simulink subsystem "PvtSubSys_VSM_LCK"  (R2020b)
settings: Solver=VariableStepAuto  StartTime=0.0  StopTime=10.0  RelTol=1e-3
values from neighbouring files (symbols this model uses):
  LCK_STATE : value not decoded    [LCK.sldd]
  P_VSM_LCK_A1 = 15.0    [LCK.sldd]
  P_VSM_LCK_AbsEspInTime = 3.0    [LCK.sldd]
  P_VSM_LCK_absLongitudeAccIn = 2.5    [LCK.sldd]
  P_VSM_LCK_absLongitudeAccOut = 3.0    [LCK.sldd]
  P_VSM_LCK_AccRateIn = 30.0    [LCK.sldd]
  P_VSM_LCK_AccRateInTime = 1.5    [LCK.sldd]
  P_VSM_LCK_AccRateOut = 80.0    [LCK.sldd]
  P_VSM_LCK_AccrPelOut = 30.0    [LCK.sldd]
  P_VSM_LCK_AccrPelRateOut = 0.0    [LCK.sldd]
  P_VSM_LCK_BrakePressIn = 3.0    [LCK.sldd]
  P_VSM_LCK_BrakePressInTime = 1.5    [LCK.sldd]
  P_VSM_LCK_BrakePressOut = 5.0    [LCK.sldd]
  P_VSM_LCK_C0 = 0.4    [LCK.sldd]
  P_VSM_LCK_DrvInputTrqValueIn = 2.0    [LCK.sldd]
  P_VSM_LCK_DrvInputTrqValueInTime = 3.0    [LCK.sldd]
  P_VSM_LCK_DrvInputTrqValueOut = 2.3    [LCK.sldd]
  P_VSM_LCK_dypreFactor = 1.0    [LCK.sldd]
  P_VSM_LCK_IdleInTime = 2.0    [LCK.sldd]
  P_VSM_LCK_LanechangeSwitch = 0.0    [LCK.sldd]
  P_VSM_LCK_LaneDouble = 1.0    [LCK.sldd]
  P_VSM_LCK_Lanewidthswitch = 1.0    [LCK.sldd]
  P_VSM_LCK_LateralAcceIn = 3.0    [LCK.sldd]
  P_VSM_LCK_LateralAcceInTime = 3.0    [LCK.sldd]
  P_VSM_LCK_LateralAcceOut = 3.5    [LCK.sldd]
  P_VSM_LCK_LCDrvInputTrqValueOut = 3.0    [LCK.sldd]
  P_VSM_LCK_LCOverrideTime = 0.6    [LCK.sldd]
  P_VSM_LCK_LCOverrideValue = 1.5    [LCK.sldd]
  P_VSM_LCK_LongitudeAccIn = 3.0    [LCK.sldd]
  P_VSM_LCK_LongitudeAccInTime = 3.0    [LCK.sldd]
  P_VSM_LCK_LongitudeAccOut = 3.5    [LCK.sldd]
  P_VSM_LCK_OverrideInTime = 3.0    [LCK.sldd]
  P_VSM_LCK_OverrideTime = 0.3    [LCK.sldd]
  P_VSM_LCK_OverrideValue = 1.2    [LCK.sldd]
  P_VSM_LCK_ParamA1 : value not decoded    [LCK.sldd]
  P_VSM_LCK_PreTime = 0.2    [LCK.sldd]
  P_VSM_LCK_State_Absesp_enable = 1.0    [LCK.sldd]
  P_VSM_LCK_State_Accpedalrate_enable = 0.0    [LCK.sldd]
  P_VSM_LCK_State_Breakpressure_enable = 1.0    [LCK.sldd]
  P_VSM_LCK_State_DriverInputTrqValue_enable = 1.0    [LCK.sldd]
  P_VSM_LCK_State_Eps_enable = 1.0    [LCK.sldd]
  P_VSM_LCK_State_ESSSts_enable = 1.0    [LCK.sldd]
  P_VSM_LCK_State_GEAR_enable = 1.0    [LCK.sldd]
  P_VSM_LCK_State_Handson_enable = 1.0    [LCK.sldd]
  P_VSM_LCK_State_IdleInTime_enable = 0.0    [LCK.sldd]
  P_VSM_LCK_State_Lane_enable = 1.0    [LCK.sldd]
  P_VSM_LCK_State_LaneChange_enable = 1.0    [LCK.sldd]
  P_VSM_LCK_State_LaneCurve_enable = 0.0    [LCK.sldd]
  P_VSM_LCK_State_LateralAcce_enable = 1.0    [LCK.sldd]
  P_VSM_LCK_State_LongitudeAcc_enable = 1.0    [LCK.sldd]
  P_VSM_LCK_State_LSMLine_enable = 1.0    [LCK.sldd]
  P_VSM_LCK_State_Overide_enable = 1.0    [LCK.sldd]
  P_VSM_LCK_State_Param_LaneCurve : value not decoded    [LCK.sldd]
  P_VSM_LCK_State_Param_LaneCurve_Offset : value not decoded    [LCK.sldd]
  P_VSM_LCK_State_Param_LaneWidth : value not decoded    [LCK.sldd]
  P_VSM_LCK_State_Param_LaneWidth_Offset : value not decoded    [LCK.sldd]
  P_VSM_LCK_State_SteerWheelAngle_enable = 1.0    [LCK.sldd]
  P_VSM_LCK_State_SteerWheelSpd_enable = 1.0    [LCK.sldd]
  P_VSM_LCK_State_TargetLaneIn_enable = 1.0    [LCK.sldd]
  P_VSM_LCK_State_TurnLight_enable = 1.0    [LCK.sldd]
  P_VSM_LCK_State_Vehspeed_enable = 1.0    [LCK.sldd]
  P_VSM_LCK_State_Yawsup_enable = 1.0    [LCK.sldd]
  P_VSM_LCK_SteerAngleSpdIn = 150.0    [LCK.sldd]
  P_VSM_LCK_SteerAngleSpdInTime = 3.0    [LCK.sldd]
  P_VSM_LCK_SteerAngleSpdOut = 200.0    [LCK.sldd]
  P_VSM_LCK_SteerWheelAngleIn = 70.0    [LCK.sldd]
  P_VSM_LCK_SteerWheelAngleInTime = 3.0    [LCK.sldd]
  P_VSM_LCK_SteerWheelAngleOut = 90.0    [LCK.sldd]
  P_VSM_LCK_T0 = 0.75    [LCK.sldd]
  P_VSM_LCK_T1 = 15.0    [LCK.sldd]
  P_VSM_LCK_TargetInSwitch = 0.0    [LCK.sldd]
  P_VSM_LCK_Warnarea1 = -0.55    [LCK.sldd]
  P_VSM_LCK_Warnarea2 = -0.35    [LCK.sldd]
  P_VSM_LCK_YawRateIn = 0.2    [LCK.sldd]
  P_VSM_LCK_YawRateInTime = 1.0    [LCK.sldd]
  P_VSM_LCK_YawRateOut = 0.25    [LCK.sldd]
undefined symbols (not defined in the file or in its folder): P_VSM_LSMC_SampleTime
libraries: simulink x275
(part 2 of 5)

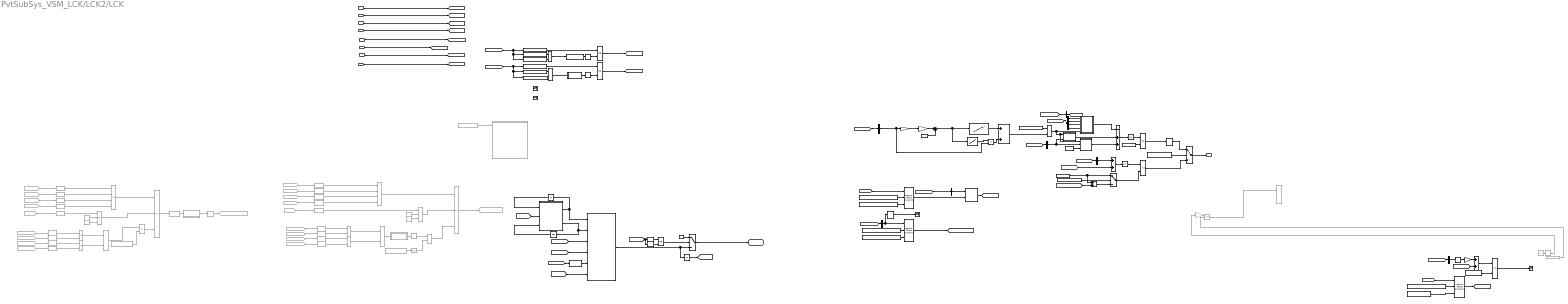
== system PvtSubSys_VSM_LCK/LCK2/LCK ==
  FLWhelDy : Inport
  FRWhelDy : Inport  Port=2
  LCKState : Inport  Port=3
  HWASts : Inport  Port=4
  LSM_LCK_CLane : Inport  Port=5
  VehSpd : Inport  Port=6
  Lane : Inport  Port=7
  TJALine : Inport  Port=8
  Abs : Abs
  Abs15 : Abs  Commented=on
  Abs16 : Abs
  Add{,2..4} (4 alike) : Sum
  Add1 : Sum  Inputs=-++
  Atan : Trigonometry  Operator=atan
  Atan2 : Trigonometry  Commented=on  Operator=atan
  Bus Selector : BusSelector  OutputSignals=LaneCurve
  Bus Selector1 : BusSelector  OutputSignals=EVI_VehicleSpd_ms
  Bus Selector2 : BusSelector  OutputSignals=EVI_Kap
  Bus Selector3 : BusSelector  OutputSignals=TJALineC2
  Bus Selector4 : BusSelector  OutputSignals=TJALineC0
  Bus Selector5 : BusSelector  OutputSignals=LDWLKAELK_LWidth
  Bus Selector6 : BusSelector  OutputSignals=TJALineC1
  Bus Selector7 : BusSelector  OutputSignals=TJALineC0,TJALineC1,TJALineC2,TJALineC3
  Compare To Constant : simulink/Logic and Bit Operations/Compare To Constant  relop===  const=5  OutDataTypeStr=boolean
  Compare To Constant1 : simulink/Logic and Bit Operations/Compare To Constant  Commented=on  relop===  const=3  OutDataTypeStr=boolean
  Compare To Constant{2,8,10,13,27..30} (8 alike) : simulink/Logic and Bit Operations/Compare To Constant  Commented=on  relop=>  const=0  OutDataTypeStr=boolean
  Compare To Constant14 : simulink/Logic and Bit Operations/Compare To Constant  Commented=on  relop=>  const=2.5  OutDataTypeStr=boolean
  Compare To Constant15 : simulink/Logic and Bit Operations/Compare To Constant  Commented=on  relop=>  const=0.5  OutDataTypeStr=boolean
  Compare To Constant{17,19,21..22,31..33,35} (8 alike) : simulink/Logic and Bit Operations/Compare To Constant  Commented=on  relop===  const=0  OutDataTypeStr=boolean
  Compare To Constant20 : simulink/Logic and Bit Operations/Compare To Constant  Commented=on  relop=<  const=2.45  OutDataTypeStr=boolean
  Compare To Constant3 : simulink/Logic and Bit Operations/Compare To Constant  Commented=on  relop=~=  const=2  OutDataTypeStr=boolean
  Compare To Constant36 : simulink/Logic and Bit Operations/Compare To Constant  Commented=on  relop=>  const=0.25  OutDataTypeStr=boolean
  Compare To Constant4 : simulink/Logic and Bit Operations/Compare To Constant  Commented=on  relop=~=  const=3  OutDataTypeStr=boolean
  Compare To Constant43 : simulink/Logic and Bit Operations/Compare To Constant  Commented=on  relop===  const=2  OutDataTypeStr=boolean
  Compare To Constant44 : simulink/Logic and Bit Operations/Compare To Constant  relop=<  const=P_VSM_LCK_Warnarea2  OutDataTypeStr=boolean
  Compare To Constant45 : simulink/Logic and Bit Operations/Compare To Constant  relop=>  const=2  OutDataTypeStr=boolean
  Compare To Constant46 : simulink/Logic and Bit Operations/Compare To Constant  relop=>=  const=P_VSM_LCK_Warnarea1  OutDataTypeStr=boolean
  Compare To Constant47 : simulink/Logic and Bit Operations/Compare To Constant  relop=<  const=P_VSM_LCK_Warnarea1  OutDataTypeStr=boolean
  Compare To Constant48 : simulink/Logic and Bit Operations/Compare To Constant  relop=<  const=P_VSM_LCK_Warnarea2  OutDataTypeStr=boolean
  Compare To Constant49 : simulink/Logic and Bit Operations/Compare To Constant  relop=>  const=2  OutDataTypeStr=boolean
  Compare To Constant5 : simulink/Logic and Bit Operations/Compare To Constant  relop===  const=6  OutDataTypeStr=boolean
  Compare To Constant50 : simulink/Logic and Bit Operations/Compare To Constant  relop=>=  const=P_VSM_LCK_Warnarea1  OutDataTypeStr=boolean
  Compare To Constant51 : simulink/Logic and Bit Operations/Compare To Constant  relop=<  const=P_VSM_LCK_Warnarea1  OutDataTypeStr=boolean
  Constant : Constant  Commented=on  Value=P_VSM_LCK_PreTime
  Constant1 : Constant  Value=1.3  OutDataTypeStr=single
  Constant10 : Constant  Value=P_VSM_LCK_A1
  Constant11 : Constant  Value=P_VSM_LCK_ParamA1
  Constant16 : Constant  Commented=on  Value=P_VSM_LCK_T1
  Constant18 : Constant  Value=P_VSM_LCK_T0
  Constant2 : Constant  Value=0
  Constant3 : Constant  Value=P_VSM_LCK_dypreFactor
  Constant4 : Constant  Value=1.6429  OutDataTypeStr=single
  Constant5 : Constant  Value=P_VSM_LCK_TargetInSwitch
  Constant6 : Constant  Commented=on  Value=P_VSM_LCK_LaneDouble
  Constant7 : Constant  Value=P_VSM_LCK_C0
  Constant8 : Constant  Commented=on  Value=P_VSM_LCK_LaneDouble
  Constant9 : Constant  Value=P_VSM_LCK_Lanewidthswitch
  Data Type Conversion1 : DataTypeConversion  Commented=on  OutDataTypeStr=double
  Data Type Conversion19 : DataTypeConversion  OutDataTypeStr=uint8
  From107 : From  Commented=on  GotoTag=Orginal_L_Lvalid
  From108 : From  Commented=on  GotoTag=Orginal_R_Lvalid
  From109 : From  Commented=on  GotoTag=Orginal_L_Revalid
  From110 : From  Commented=on  GotoTag=Orginal_R_Revalid
  From111 : From  Commented=on  GotoTag=L
  From112 : From  Commented=on  GotoTag=Orginal_R_Lvalid
  From113 : From  Commented=on  GotoTag=Orginal_L_Revalid
  From114 : From  Commented=on  GotoTag=Orginal_R_Revalid
  From36 : From  Commented=on  GotoTag=L
  From38 : From  Commented=on  GotoTag=Left_LaneValid
  From39 : From  Commented=on  GotoTag=Right_LaneValid
  From41 : From  Commented=on  GotoTag=Left_ReValid
  From43 : From  Commented=on  GotoTag=Right_ReValid
  From58 : From  Commented=on  GotoTag=Orginal_L_Lvalid
  From59 : From  Commented=on  GotoTag=Left_LaneValid
  From60 : From  Commented=on  GotoTag=Right_LaneValid
  From61 : From  Commented=on  GotoTag=Left_ReValid
  From62 : From  Commented=on  GotoTag=Right_ReValid
  Gain : Gain  Gain=57.3
  Gain1 : Gain  Gain=1.03
  Gain3 : Gain  Gain=3.6
  Gain4 : Gain  Commented=on  Gain=57.3
  Goto1 : Goto  Commented=on  GotoTag=LCK_Line_Out
  Goto8 : Goto  Commented=on  GotoTag=LCK_Line_In
  Lane_Width_table1 : Constant  Value=P_VSM_LCK_State_Param_LaneWidth
  Lane_Width_table2 : Constant  Value=P_VSM_LCK_State_Param_LaneCurve
  Lane_Width_table3 : Constant  Value=P_VSM_LCK_State_Param_LaneCurve
  Logical Operator : Logic  AllPortsSameDT=off  OutDataTypeStr=boolean
  Logical Operator{1,3,16..17,23,48} (6 alike) : Logic  Commented=on  AllPortsSameDT=off  OutDataTypeStr=boolean
  Logical Operator12 : Logic  Commented=on  Operator=OR  AllPortsSameDT=off  OutDataTypeStr=boolean
  Logical Operator13 : Logic  Commented=on  Operator=OR  AllPortsSameDT=off  OutDataTypeStr=boolean
  Logical Operator14 : Logic  Commented=on  Operator=OR  Inputs=4  AllPortsSameDT=off  OutDataTypeStr=boolean
  Logical Operator15 : Logic  Commented=on  Inputs=3  AllPortsSameDT=off  OutDataTypeStr=boolean
  Logical Operator18 : Logic  Operator=OR  AllPortsSameDT=off  OutDataTypeStr=boolean
  Logical Operator19 : Logic  AllPortsSameDT=off  OutDataTypeStr=boolean
  Logical Operator2 : Logic  Commented=on  Operator=OR  Inputs=3  AllPortsSameDT=off  OutDataTypeStr=boolean
  Logical Operator20 : Logic  Operator=OR  AllPortsSameDT=off  OutDataTypeStr=boolean
  Logical Operator21 : Logic  Commented=on  Operator=OR  AllPortsSameDT=off  OutDataTypeStr=boolean
  Logical Operator22 : Logic  Commented=on  Inputs=4  AllPortsSameDT=off  OutDataTypeStr=boolean
  Logical Operator37 : Logic  Commented=on  Operator=NOT  AllPortsSameDT=off  OutDataTypeStr=boolean
  Logical Operator4 : Logic  Operator=OR  AllPortsSameDT=off  OutDataTypeStr=boolean
  Logical Operator42 : Logic  Commented=on  Operator=OR  Inputs=3  AllPortsSameDT=off  OutDataTypeStr=boolean
  Logical Operator43 : Logic  Commented=on  Inputs=3  AllPortsSameDT=off  OutDataTypeStr=boolean
  Lookup Table Dynamic1 : simulink/Lookup Tables/Lookup Table Dynamic  LookUpMeth=Interpolation-Use End Values  OutDataType=fixdt('double')  OutScaling=[]  OutputDataTypeScalingMode=Specify via dialog  OutDataTypeStr=double  DoSatur=off
  Lookup Table Dynamic2 : simulink/Lookup Tables/Lookup Table Dynamic  LookUpMeth=Interpolation-Use End Values  OutDataType=fixdt('double')  OutScaling=[]  OutputDataTypeScalingMode=Specify via dialog  OutDataTypeStr=double  DoSatur=off
  Lookup Table Dynamic3 : simulink/Lookup Tables/Lookup Table Dynamic  LookUpMeth=Interpolation-Use End Values  OutDataType=fixdt('double')  OutScaling=[]  OutputDataTypeScalingMode=Specify via dialog  OutDataTypeStr=double  DoSatur=off
  MATLAB Function : MATLAB Function  TreatAsAtomicUnit=on
  MATLAB Function1 : MATLAB Function  Commented=on  TreatAsAtomicUnit=on
  MATLAB Function2 : MATLAB Function  TreatAsAtomicUnit=on
  MATLAB Function3 : MATLAB Function  TreatAsAtomicUnit=on
  MATLAB Function4 : MATLAB Function  TreatAsAtomicUnit=on
  MATLAB Function5 : MATLAB Function  TreatAsAtomicUnit=on
  MATLAB Function6 : MATLAB Function  TreatAsAtomicUnit=on
  Offset1 : Constant  Value=P_VSM_LCK_State_Param_LaneWidth_Offset
  Offset2 : Constant  Value=P_VSM_LCK_State_Param_LaneCurve_Offset
  Product : Product
  Product2 : Product
  Relational Operator : RelationalOperator  Commented=on  Operator=<=  OutDataTypeStr=boolean  RndMeth=Simplest
  Relational Operator1 : RelationalOperator  Operator=<=  OutDataTypeStr=boolean  RndMeth=Simplest
  Relational Operator2 : RelationalOperator  Operator=<=  OutDataTypeStr=boolean  RndMeth=Simplest
  Relational Operator5 : RelationalOperator  Operator=<=  OutDataTypeStr=boolean  RndMeth=Simplest
  Signal Copy : SignalConversion  OverrideOpt=off
  Signal Copy1 : SignalConversion  OverrideOpt=off
  Subsystem1 : Subsystem  Commented=on  mask{Ts=P_VSM_LSMC_SampleTime, Max=10}
      mask prompts: Ts "Sample Time:"; Max "Max Limit:"
      mask Display:
      | Ts=get_param(gcb,'Ts');
      | Max=get_param(gcb,'Max');
      | disp(['Ts:' Ts '\n' 'Max:' Max ]);
  Subsystem2 : Subsystem  mask{Ts=P_VSM_LSMC_SampleTime, Max=10}
      mask prompts: Ts "Sample Time:"; Max "Max Limit:"
      mask Display:
      | Ts=get_param(gcb,'Ts');
      | Max=get_param(gcb,'Max');
      | disp(['Ts:' Ts '\n' 'Max:' Max ]);
  Subsystem3 : Subsystem  mask{Ts=P_VSM_LSMC_SampleTime, Max=10}
      mask prompts: Ts "Sample Time:"; Max "Max Limit:"
      mask Display:
      | Ts=get_param(gcb,'Ts');
      | Max=get_param(gcb,'Max');
      | disp(['Ts:' Ts '\n' 'Max:' Max ]);
  Subsystem5 : Subsystem  Commented=on  mask{Ts=P_VSM_LSMC_SampleTime, Max=10}
      mask prompts: Ts "Sample Time:"; Max "Max Limit:"
      mask Display:
      | Ts=get_param(gcb,'Ts');
      | Max=get_param(gcb,'Max');
      | disp(['Ts:' Ts '\n' 'Max:' Max ]);
  Sum : Sum  Inputs=|++
  Switch : Switch  Criteria=u2 > Threshold
  Switch1 : Switch  Criteria=u2 > Threshold
  Switch2 : Switch  Criteria=u2 > Threshold
  Terminator{,1..3} (4 alike) : Terminator
  Unit Delay1 : UnitDelay  SampleTime=-1  HasFrameUpgradeWarning=on
  Unit Delay2 : UnitDelay  SampleTime=-1  HasFrameUpgradeWarning=on
  Unit Delay7 : UnitDelay  SampleTime=-1  HasFrameUpgradeWarning=on
  preDisMinTable : Lookup_n-D  NumberOfTableDimensions=1  BreakpointsForDimension1=[0 5 10 15 20 25 30 35 40 60 80 90 100 110 120 140]  Table=[8 9 10 11 12 13 14 15 17 22 28 31 35 38 42 49]  ExtrapMethod=Clip  InternalRulePriority=Speed  RndMeth=Simplest  InputSameDT=on
  tDeltaEpsTable : Lookup_n-D  NumberOfTableDimensions=1  BreakpointsForDimension1=[0 5 10 15 20 25 30 35 40 60 80 90 100 110 120 140]  Table=[0.8 0.8 0.77803 0.75258 0.71864 0.65924 0.5447 0.45773 0.38348 0.2 0.2 0.2 0.20106 0.2 0.2 0.2]  ExtrapMethod=Clip  InternalRulePriority=Speed  RndMeth=Simplest  InputSameDT=on
  LCKWarning : Outport
  LCK_TargetLaneIn : Outport  Port=2
  wires:
  Abs/1 -> Relational Operator1/1  "VSM_LCK_d0"
  Relational Operator2/1 -> Terminator3/1  "VSM_LCK_TargetLaneIn_A1"
  Lookup Table Dynamic2/1 -> [headingangle_Offset]
  Constant11/1 -> Lookup Table Dynamic2/3
  Lane_Width_table3/1 -> Lookup Table Dynamic2/2
  [LaneCurve] -> Lookup Table Dynamic2/1
  Constant10/1 -> Relational Operator2/2
  Add4/1 -> Relational Operator2/1
  [headingangle_Offset] -> Add4/2
  Gain/1 -> Add4/1
  Bus Selector6/1 -> Atan/1  "<TJALineC1>"
  [TJALine] -> Bus Selector6/1
  Atan/1 -> Gain/1
  Add3/1 -> Switch1/3
  Switch1/1 -> Relational Operator1/2
  [P_VSM_LKA_LaneWidth_Offset] -> Add3/2
  Constant9/1 -> Switch1/2
  Signal Copy1/1 -> Terminator2/1  "VSM_LCK_Lanewidth"
  [LSM_LCK_CLane] -> Bus Selector5/1
  Lookup Table Dynamic1/1 -> [P_VSM_LKA_LaneWidth_Offset]  "VSM_LCK_LaneWidth_offset"
  Bus Selector5/1 -> Lookup Table Dynamic1/1, Signal Copy1/1  "<LDWLKAELK_LWidth>"
  Offset1/1 -> Lookup Table Dynamic1/3
  Lane_Width_table1/1 -> Lookup Table Dynamic1/2
  Constant7/1 -> Add3/1, Switch1/1
  Relational Operator1/1 -> Switch/3  "VSM_LCK_TargetLaneIn2"
  Add2/1 -> Abs/1
  [TJALine] -> Bus Selector4/1
  Bus Selector4/1 -> Add2/1  "<TJALineC0>"
  [LaneCurve_Offset] -> Add2/2  "VSM_LCK_LaneCure_Offset"
  Switch/1 -> LCK_TargetLaneIn/1
  MATLAB Function6/1(Offset) -> [LaneCurve_Offset]
  Bus Selector3/1 -> MATLAB Function6/1(T_A2)  "<TJALineC2>"
  [TJALine] -> Bus Selector3/1
  Lane_Width_table2/1 -> Lookup Table Dynamic3/2
  Offset2/1 -> Lookup Table Dynamic3/3
  [LaneCurve] -> Lookup Table Dynamic3/1  "VSM_LCK_LaneCure"
  Lookup Table Dynamic3/1 -> MATLAB Function6/2(LaneCurveOffset)
  Constant5/1 -> Switch/2
  Signal Copy/1 -> Switch/1
  Relational Operator5/1 -> Signal Copy/1  "VSM_LCK_TargetLaneIn"
  Bus Selector/1 -> [LaneCurve]  "<LaneCurve>"
  Bus Selector2/1 -> MATLAB Function/2(kap), MATLAB Function4/2(kap)  "<EVI_Kap>"
  Add/1 -> Product2/2  "VSM_LCK_preDis"
  [Lane] -> Bus Selector2/1
  tDeltaEpsTable/1 -> Product/1
  Sum/1 -> tDeltaEpsTable/1, preDisMinTable/1
  preDisMinTable/1 -> Add/1
  Product/1 -> Add/2
  Gain1/1 -> Sum/1
  Constant1/1 -> Sum/2
  Gain3/1 -> Gain1/1
  Compare To Constant5/1 -> Logical Operator4/2
  Compare To Constant/1 -> Logical Operator4/1
  [HWASts] -> Compare To Constant/1, Compare To Constant5/1
  Bus Selector1/1 -> Gain3/1, Product/2  "<EVI_VehicleSpd_ms>"
  VehSpd/1 -> [VehSpd]
  Constant/1 -> MATLAB Function1/1(tCycle)
  ? -> Terminator1/1
  ? -> Terminator/1
  ? -> Abs15/1
  Add1/1 -> Abs16/1
  [LSM_LCK_CLane] -> Bus Selector/1
  LSM_LCK_CLane/1 -> [LSM_LCK_CLane]
  Abs16/1 -> Relational Operator5/1
  Gain4/1 -> Relational Operator/1
  Relational Operator/1 -> Logical Operator48/1  "VSM_LCK_TargetLaneIn_A1"
  Abs15/1 -> Atan2/1
  Constant16/1 -> Relational Operator/2
  Atan2/1 -> Gain4/1
  Constant18/1 -> Relational Operator5/2
  Compare To Constant15/1 -> Goto8/1
  Logical Operator2/1 -> Goto1/1
  Logical Operator1/1 -> Subsystem5/1(In1)
  Compare To Constant2/1 -> Logical Operator14/1
  Compare To Constant28/1 -> Logical Operator12/2
  Compare To Constant13/1 -> Logical Operator14/4
  Compare To Constant4/1 -> Logical Operator43/3
  Compare To Constant17/1 -> Logical Operator22/3
  Logical Operator3/1 -> Logical Operator21/1
  Compare To Constant10/1 -> Logical Operator14/3
  From113/1 -> Compare To Constant32/1
  Logical Operator43/1 -> Logical Operator2/2
  Logical Operator12/1 -> Logical Operator3/1
  Compare To Constant32/1 -> Logical Operator16/2
  Compare To Constant43/1 -> Logical Operator42/2
  Compare To Constant3/1 -> Logical Operator43/2
  From36/1 -> Compare To Constant20/1
  Compare To Constant33/1 -> Logical Operator17/1
  From58/1 -> Compare To Constant31/1
  Compare To Constant20/1 -> Logical Operator43/1
  Subsystem1/1(Out1) -> Compare To Constant15/1
  From61/1 -> Compare To Constant17/1
  Logical Operator42/1 -> Logical Operator15/2
  From107/1 -> Compare To Constant27/1
  Data Type Conversion1/1 -> Subsystem1/1(In1)
  From114/1 -> Compare To Constant35/1
  From60/1 -> Compare To Constant22/1
  Compare To Constant36/1 -> Logical Operator23/1
  Compare To Constant27/1 -> Logical Operator12/1
  From111/1 -> Compare To Constant14/1
  Logical Operator23/1 -> Logical Operator2/3
  Constant8/1 -> Logical Operator37/1
  Compare To Constant8/1 -> Logical Operator14/2
  From109/1 -> Compare To Constant28/1
  ? -> Compare To Constant3/1, Compare To Constant4/1
  From43/1 -> Compare To Constant13/1
  From41/1 -> Compare To Constant10/1
  Compare To Constant14/1 -> Logical Operator42/1  "VSM_LCK_LWidth_valid"
  From39/1 -> Compare To Constant8/1
  Compare To Constant29/1 -> Logical Operator13/1
  Logical Operator21/1 -> Logical Operator15/3
  Compare To Constant21/1 -> Logical Operator22/1
  Compare To Constant1/1 -> Logical Operator42/3
  Logical Operator15/1 -> Data Type Conversion1/1
  Logical Operator14/1 -> Logical Operator15/1  "VSM_LCK_Lane_valid"
  From62/1 -> Compare To Constant19/1
  From108/1 -> Compare To Constant29/1
  Compare To Constant30/1 -> Logical Operator13/2
  From110/1 -> Compare To Constant30/1
  Logical Operator13/1 -> Logical Operator3/2
  Constant6/1 -> Logical Operator21/2
  Compare To Constant19/1 -> Logical Operator22/4
  Logical Operator17/1 -> Logical Operator1/2
  Compare To Constant31/1 -> Logical Operator16/1
  From112/1 -> Compare To Constant33/1
  Logical Operator16/1 -> Logical Operator1/1
  Compare To Constant35/1 -> Logical Operator17/2
  Subsystem5/1(Out1) -> Compare To Constant36/1
  From38/1 -> Compare To Constant2/1
  Logical Operator22/1 -> Logical Operator2/1
  From59/1 -> Compare To Constant21/1
  Compare To Constant22/1 -> Logical Operator22/2
  Logical Operator37/1 -> Logical Operator23/2
  FLWhelDy/1 -> [FLWhelDy]
  Compare To Constant48/1 -> Logical Operator19/1
  Compare To Constant46/1 -> Logical Operator/2
  Subsystem3/1(Out1) -> Compare To Constant49/1
  Logical Operator19/1 -> Subsystem3/1(In1)
  Compare To Constant51/1 -> Logical Operator20/1
  Subsystem2/1(Out1) -> Compare To Constant45/1
  Compare To Constant44/1 -> Logical Operator/1
  Compare To Constant45/1 -> Logical Operator18/2
  Compare To Constant47/1 -> Logical Operator18/1
  Compare To Constant50/1 -> Logical Operator19/2
  Compare To Constant49/1 -> Logical Operator20/2
  Logical Operator/1 -> Subsystem2/1(In1)
  FRWhelDy/1 -> [FRWhelDy]
  LCKState/1 -> [LCKState]
  HWASts/1 -> [HWASts]
  [FLWhelDy] -> Compare To Constant46/1, Compare To Constant44/1, Compare To Constant47/1
  [FRWhelDy] -> Compare To Constant50/1, Compare To Constant48/1, Compare To Constant51/1
  Logical Operator18/1 -> [LCK_LeftWarning]
  Logical Operator20/1 -> [LCK_RightWarning]
  [LCK_LeftWarning] -> MATLAB Function2/3(LCK_LeftWarn)
  MATLAB Function2/1(LCKWarning) -> Unit Delay1/1, Switch2/3
  [LCKWarning] -> MATLAB Function2/6(LCKWarningK1)
  [LCKWarning] -> MATLAB Function3/2(LCKWarning)
  Switch2/1 -> LCKWarning/1  "VSM_LCK_Warning"
  Constant2/1 -> Switch2/1
  MATLAB Function3/1(OutCount) -> Unit Delay2/1, MATLAB Function2/1(OutCount)
  Logical Operator4/1 -> Switch2/2
  [LCKState] -> Data Type Conversion19/1
  Unit Delay2/1 -> MATLAB Function3/1(data)
  MATLAB Function3/2(InCount) -> Unit Delay7/1, MATLAB Function2/2(InCount)
  Unit Delay1/1 -> [LCKWarning]
  [LCK_RightWarning] -> MATLAB Function2/4(LCK_RightWarn)
  Unit Delay7/1 -> MATLAB Function3/3(data1)
  Data Type Conversion19/1 -> MATLAB Function2/5(LCKState)
  Lane/1 -> [Lane]
  [Lane] -> Bus Selector1/1
  MATLAB Function/1(dy_pre) -> Add1/2  "VSM_LCK_dypre"
  Constant3/1 -> Product2/1
  Product2/1 -> MATLAB Function4/1(predis), MATLAB Function/1(preDis), MATLAB Function5/5(predis)
  Constant4/1 -> MATLAB Function4/3(Dx)
  MATLAB Function4/1(offset) -> Add1/3  "VSM_LCK_dypreoffset"
  MATLAB Function5/1(dy0) -> Add1/1  "VSM_LCK_dy0"
  TJALine/1 -> [TJALine]
  [TJALine] -> Bus Selector7/1
  Bus Selector7/1 -> MATLAB Function5/1(A0)  "<TJALineC0>"
  Bus Selector7/2 -> MATLAB Function5/2(A1)  "<TJALineC1>"
  Bus Selector7/3 -> MATLAB Function5/3(A2)  "<TJALineC2>"
  Bus Selector7/4 -> MATLAB Function5/4(A3)  "<TJALineC3>"
